simulink model "gm_Test_DOA"  (R2020b)
settings: Solver=ode4  StartTime=0.0  StopTime=0.16  RelTol=1e-3
undefined symbols (not defined in the file or in its folder): f_range, FFT_LENGTH, Sampling_rate
libraries: dsphdlmathfun x4, dsphdlxfrm x4, hdlsllib x1
(part 2 of 2)

== system gm_Test_DOA/Maximum Hydro Ref/Subsystem ==
  Enable/Reset : Inport  OutDataTypeStr=boolean  PortDimensions=1  SampleTime=1e-07
  Add : Sum
  Data Type Conversion1 : DataTypeConversion  OutDataTypeStr=uint16  RndMeth=Nearest
  Delay : Delay  DelayLength=1  InitialCondition=0  UseCircularBuffer=on
  Product2 : Product
  Count : Outport  VectorParamsAs1DForOutWhenUnconnected=off
  wires:
  Enable/Reset/1 -> Product2/1, Add/1
  Add/1 -> Product2/2
  Data Type Conversion1/1 -> Add/2
  Delay/1 -> Data Type Conversion1/1, Count/1
  Product2/1 -> Delay/1

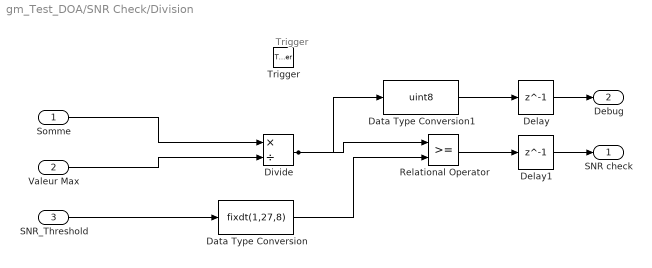
== system gm_Test_DOA/SNR Check/Division ==
  note: Trigger
  Somme : Inport  OutDataTypeStr=fixdt(1, 27, 8)  PortDimensions=1
  " Valeur Max" : Inport  Port=2  OutDataTypeStr=fixdt(1, 18, 0)  PortDimensions=1
  SNR_Threshold : Inport  Port=3  OutDataTypeStr=uint8  PortDimensions=1
  Trigger : TriggerPort  VariantControl=(inherit)  PortDimensions=1  OutDataTypeStr=boolean
  Data Type Conversion : DataTypeConversion  OutDataTypeStr=fixdt(1,27,8)
  Data Type Conversion1 : DataTypeConversion  OutDataTypeStr=uint8
  Delay : Delay  DelayLength=1
  Delay1 : Delay  DelayLength=1
  Divide : Product  Inputs=*/  RndMeth=Zero  SaturateOnIntegerOverflow=on
  Relational Operator : RelationalOperator  OutDataTypeStr=boolean  RndMeth=Simplest
  SNR check : Outport  InitialOutput=0  VectorParamsAs1DForOutWhenUnconnected=off
  Debug : Outport  Port=2  InitialOutput=0  VectorParamsAs1DForOutWhenUnconnected=off
  wires:
  Somme/1 -> Divide/1
  " Valeur Max"/1 -> Divide/2
  SNR_Threshold/1 -> Data Type Conversion/1
  Data Type Conversion/1 -> Relational Operator/2
  Data Type Conversion1/1 -> Delay/1
  Delay/1 -> Debug/1
  Delay1/1 -> SNR check/1
  Divide/1 -> Relational Operator/1, Data Type Conversion1/1
  Relational Operator/1 -> Delay1/1

== system gm_Test_DOA/FFTs/Trigger/SampleHold ==
  Trigger : Inport  OutDataTypeStr=boolean  PortDimensions=1  SampleTime=1e-07
  In2 : Inport  Port=2  OutDataTypeStr=boolean  PortDimensions=1  SampleTime=1e-07
  Sample and Hold : Subsystem  mask(Sample and Hold){trig=Rising edge, initCond=double(0), latchinput=off}
      mask prompts: trig "Trigger type:"; initCond "Initial condition:"; latchinput "Latch (buffer) input"
      mask help: Sample and hold the input signal. If Latch (buffer) input is selected, then this block produces the value of the input from the previous time step.
      mask init: same as gm_Test_DOA/Maximum Hydro 1/SampleHold/Sample and Hold
      mask Help: eval('blocksethelp');
      mask TypeOptions trig: Rising edge | Falling edge | Either edge
      mask Display: disp('S/H')
  " " : Outport
  wires:
  Trigger/1 -> Sample and Hold/Trigger
  In2/1 -> Sample and Hold/1(In)
  Sample and Hold/1(" ") -> " "/1

== system gm_Test_DOA/Maximum Hydro 1/SampleHold/Sample and Hold ==
  note: Trigger
  In : Inport  OutDataTypeStr=fixdt(1, 18, 0)
  Trigger : TriggerPort  TriggerType=falling  VariantControl=(inherit)  OutDataTypeStr=boolean
  " " : Outport  InitialOutput=0
  wires:
  In/1 -> " "/1

== system gm_Test_DOA/Maximum Hydro 1/SampleHold5/Sample and Hold ==
  note: Trigger
  In : Inport  OutDataTypeStr=fixdt(1, 20, 17)
  Trigger : TriggerPort  TriggerType=falling  VariantControl=(inherit)  OutDataTypeStr=boolean
  " " : Outport  InitialOutput=0
  wires:
  In/1 -> " "/1

== system gm_Test_DOA/Maximum Hydro 1/SampleHold6/Sample and Hold ==
  note: Trigger
  In : Inport  OutDataTypeStr=fixdt(1, 20, 17)
  Trigger : TriggerPort  TriggerType=falling  VariantControl=(inherit)  OutDataTypeStr=boolean
  " " : Outport  InitialOutput=0
  wires:
  In/1 -> " "/1

== system gm_Test_DOA/Maximum Hydro 2/SampleHold/Sample and Hold ==
  note: Trigger
  In : Inport  OutDataTypeStr=fixdt(1, 18, 0)
  Trigger : TriggerPort  TriggerType=falling  VariantControl=(inherit)  OutDataTypeStr=boolean
  " " : Outport  InitialOutput=0
  wires:
  In/1 -> " "/1

== system gm_Test_DOA/Maximum Hydro 2/SampleHold5/Sample and Hold ==
  note: Trigger
  In : Inport  OutDataTypeStr=fixdt(1, 20, 17)
  Trigger : TriggerPort  TriggerType=falling  VariantControl=(inherit)  OutDataTypeStr=boolean
  " " : Outport  InitialOutput=0
  wires:
  In/1 -> " "/1

== system gm_Test_DOA/Maximum Hydro 2/SampleHold6/Sample and Hold ==
  note: Trigger
  In : Inport  OutDataTypeStr=fixdt(1, 20, 17)
  Trigger : TriggerPort  TriggerType=falling  VariantControl=(inherit)  OutDataTypeStr=boolean
  " " : Outport  InitialOutput=0
  wires:
  In/1 -> " "/1

== system gm_Test_DOA/Maximum Hydro 3/SampleHold/Sample and Hold ==
  note: Trigger
  In : Inport  OutDataTypeStr=fixdt(1, 18, 0)
  Trigger : TriggerPort  TriggerType=falling  VariantControl=(inherit)  OutDataTypeStr=boolean
  " " : Outport  InitialOutput=0
  wires:
  In/1 -> " "/1

== system gm_Test_DOA/Maximum Hydro 3/SampleHold5/Sample and Hold ==
  note: Trigger
  In : Inport  OutDataTypeStr=fixdt(1, 20, 17)
  Trigger : TriggerPort  TriggerType=falling  VariantControl=(inherit)  OutDataTypeStr=boolean
  " " : Outport  InitialOutput=0
  wires:
  In/1 -> " "/1

== system gm_Test_DOA/Maximum Hydro 3/SampleHold6/Sample and Hold ==
  note: Trigger
  In : Inport  OutDataTypeStr=fixdt(1, 20, 17)
  Trigger : TriggerPort  TriggerType=falling  VariantControl=(inherit)  OutDataTypeStr=boolean
  " " : Outport  InitialOutput=0
  wires:
  In/1 -> " "/1

== system gm_Test_DOA/Maximum Hydro Ref/SampleHold/Sample and Hold ==
  note: Trigger
  In : Inport  OutDataTypeStr=fixdt(1, 18, 0)
  Trigger : TriggerPort  TriggerType=falling  VariantControl=(inherit)  OutDataTypeStr=boolean
  " " : Outport  InitialOutput=0
  wires:
  In/1 -> " "/1

== system gm_Test_DOA/Maximum Hydro Ref/SampleHold2/Sample and Hold ==
  note: Trigger
  In : Inport  OutDataTypeStr=fixdt(1, 18, 0)
  Trigger : TriggerPort  TriggerType=falling  VariantControl=(inherit)  OutDataTypeStr=boolean
  " " : Outport  InitialOutput=0
  wires:
  In/1 -> " "/1

== system gm_Test_DOA/Maximum Hydro Ref/SampleHold3/Sample and Hold ==
  note: Trigger
  In : Inport  OutDataTypeStr=fixdt(0, 17, 0)
  Trigger : TriggerPort  TriggerType=falling  VariantControl=(inherit)  OutDataTypeStr=boolean
  " " : Outport  InitialOutput=0
  wires:
  In/1 -> " "/1

== system gm_Test_DOA/Maximum Hydro Ref/SampleHold4/Sample and Hold ==
  note: Trigger
  In : Inport  OutDataTypeStr=fixdt(0, 17, 0)
  Trigger : TriggerPort  TriggerType=falling  VariantControl=(inherit)  OutDataTypeStr=boolean
  " " : Outport  InitialOutput=0
  wires:
  In/1 -> " "/1

== system gm_Test_DOA/Maximum Hydro Ref/SampleHold5/Sample and Hold ==
  note: Trigger
  In : Inport  OutDataTypeStr=fixdt(1, 20, 17)
  Trigger : TriggerPort  TriggerType=falling  VariantControl=(inherit)  OutDataTypeStr=boolean
  " " : Outport  InitialOutput=0
  wires:
  In/1 -> " "/1

== system gm_Test_DOA/Maximum Hydro Ref/SampleHold6/Sample and Hold ==
  note: Trigger
  In : Inport  OutDataTypeStr=fixdt(1, 20, 17)
  Trigger : TriggerPort  TriggerType=falling  VariantControl=(inherit)  OutDataTypeStr=boolean
  " " : Outport  InitialOutput=0
  wires:
  In/1 -> " "/1

== system gm_Test_DOA/FFTs/Trigger/SampleHold/Sample and Hold ==
  note: Trigger
  In : Inport  OutDataTypeStr=boolean
  Trigger : TriggerPort  VariantControl=(inherit)  OutDataTypeStr=boolean
  " " : Outport  InitialOutput=0
  wires:
  In/1 -> " "/1
